simulink model "circuit"  (Simulink 7.5)
settings: Solver=ode45  StartTime=0.0  StopTime=2  RelTol=1e-3
libraries: powerlib x12, powerlib_extras x1
settings Model: Creator=Singhal  LastModifiedBy=Singhal

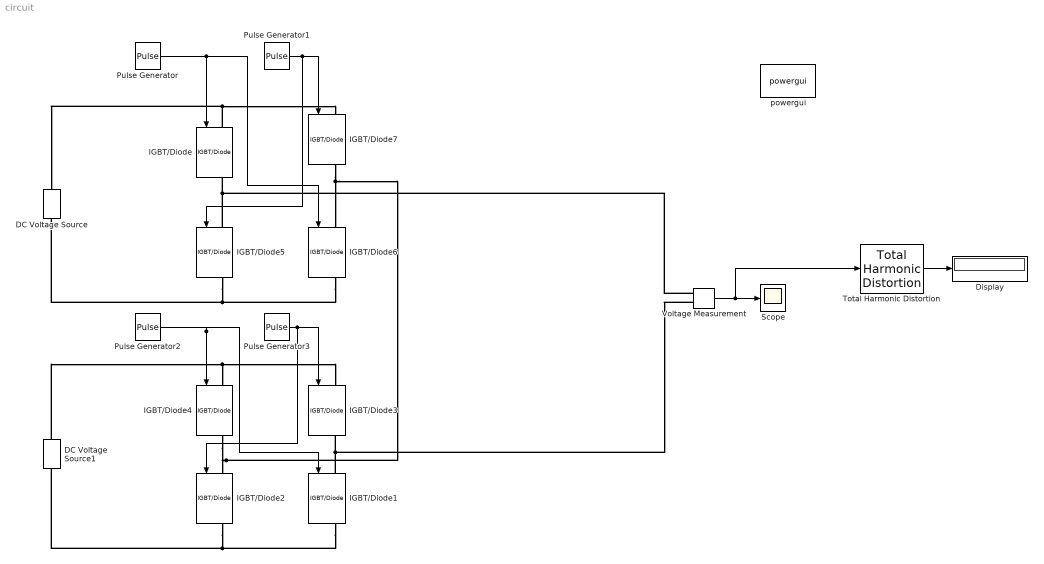
== system circuit ==
  DC Voltage Source : powerlib/Electrical Sources/DC Voltage Source  DialogController=POWERSYS.PowerSysDialog  SystemSampleTime=-1  Amplitude=100  Measurements=None
  DC Voltage Source1 : powerlib/Electrical Sources/DC Voltage Source  DialogController=POWERSYS.PowerSysDialog  SystemSampleTime=-1  Amplitude=100  Measurements=None
  Display : Display
  IGBT/Diode{,1..7} (8 alike) : powerlib/Power Electronics/IGBT//Diode  DialogController=POWERSYS.PowerSysDialog  SystemSampleTime=-1  Ron=1e-3  Rs=1e5  Cs=inf  Measurements=on
  Pulse Generator : DiscretePulseGenerator  PulseType=Time based  Amplitude=1  Period=0.02  PulseWidth=50  PhaseDelay=0  SampleTime=1
  Pulse Generator1 : DiscretePulseGenerator  PulseType=Time based  Amplitude=1  Period=0.02  PulseWidth=50  PhaseDelay=0.02/3  SampleTime=1
  Pulse Generator2 : DiscretePulseGenerator  PulseType=Time based  Amplitude=1  Period=0.02  PulseWidth=100/7  PhaseDelay=0.02/9  SampleTime=1
  Pulse Generator3 : DiscretePulseGenerator  PulseType=Time based  Amplitude=1  Period=0.02  PulseWidth=100/7  PhaseDelay=0.01+(0.02/9)  SampleTime=1  VectorParams1D=off
  Scope : Scope
  Total Harmonic Distortion : powerlib_extras/Measurements/Total Harmonic Distortion  DialogController=POWERSYS.PowerSysDialog  SystemSampleTime=-1  f1=60
  Voltage Measurement : powerlib/Measurements/Voltage Measurement  DialogController=POWERSYS.PowerSysDialog  SystemSampleTime=-1  PhasorSimulation=off  OutputType=Complex  PSBequivalent=0
  powergui : powerlib/powergui  Priority=1  SystemSampleTime=-1  SimulationMode=Continuous  SampleTime=50e-6  frequency=60  SPID=off  DisableSnubberDevices=off  DisableRonSwitches=off  DisableVfSwitches=off  SwTol=0  Interpol=off  frequencyindice=0  echomessages=off  HookPort=off  DisplayEquations=off  FunctionMessages=off  EnableUseOfTLC=off  x0status=blocks  RestoreLinks=warning  ResistiveCurrentMeasurement=off  Ylog=off  Xlog=on  ShowGrid=off  save=off  variable=ZData  ZoomFFT=off  StartTime=0.0  cycles=1  DisplayStyle=1  FreqAxis=off  MaxFrequency=1000  frequencyindicesteady=1  display=off  methode=off
  wires:
  Pulse Generator/1 -> IGBT/Diode/1, IGBT/Diode6/1
  Pulse Generator1/1 -> IGBT/Diode7/1, IGBT/Diode5/1
  Voltage Measurement/1 -> Scope/1, Total Harmonic Distortion/1
  Pulse Generator2/1 -> IGBT/Diode4/1, IGBT/Diode1/1
  Pulse Generator3/1 -> IGBT/Diode3/1, IGBT/Diode2/1
  Total Harmonic Distortion/1 -> Display/1
  connections:
  IGBT/Diode/LConn1 -- DC Voltage Source/RConn1 -- IGBT/Diode7/LConn1
  Voltage Measurement/LConn2 -- IGBT/Diode1/LConn1 -- IGBT/Diode3/RConn1
  Voltage Measurement/LConn1 -- IGBT/Diode5/LConn1 -- IGBT/Diode/RConn1
  IGBT/Diode6/RConn1 -- DC Voltage Source/LConn1 -- IGBT/Diode5/RConn1
  DC Voltage Source1/RConn1 -- IGBT/Diode3/LConn1 -- IGBT/Diode4/LConn1
  IGBT/Diode1/RConn1 -- DC Voltage Source1/LConn1 -- IGBT/Diode2/RConn1
  IGBT/Diode7/RConn1 -- IGBT/Diode6/LConn1 -- IGBT/Diode2/LConn1 -- IGBT/Diode4/RConn1
